simulink model "CE"  (R2021a)
settings: Solver=VariableStepAuto  StartTime=0.0  StopTime=10.0  RelTol=1e-3
(part 1 of 2)
settings Model: Creator=MSI-NB  LastModifiedBy=MSI-NB

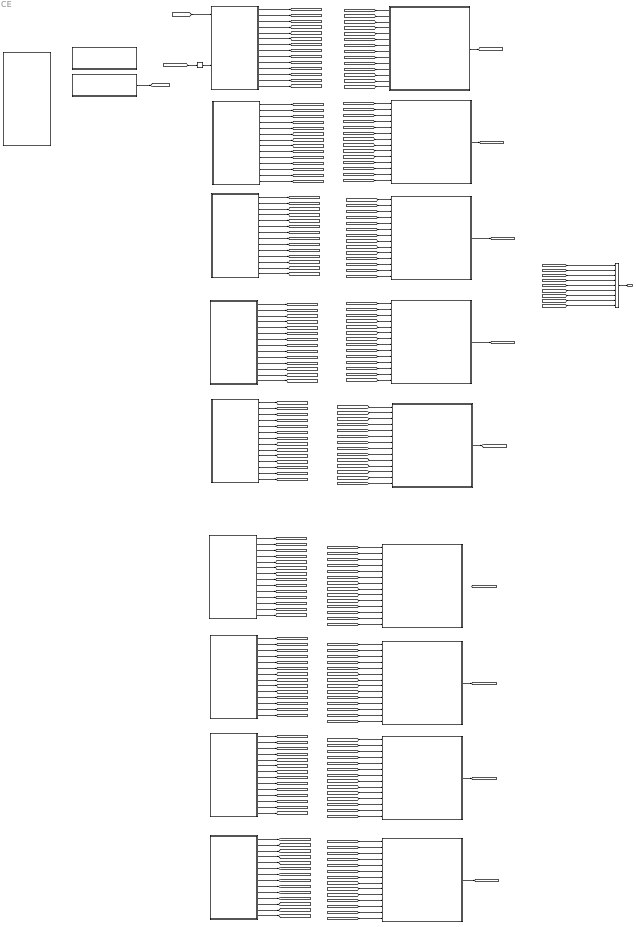
== system CE ==
  Construction : Subsystem
  Construction1 : Subsystem
  ConstructionScenarioCodition : Subsystem
  CruiseOnLane : Subsystem
  CruiseOnLaneScenarioCodition : Subsystem
  Curve : Subsystem
  CurveSenirioConditon : Subsystem
  CutinObjDengerCal : Subsystem
  ILC : Subsystem
  ILCScenarioCodition : Subsystem
  LaneChange : Subsystem
  LaneChangeScenarioCondition : Subsystem
  Memory : Memory
  MergeScenarioCodition : Subsystem
  Min : MinMax  Inputs=9
  Ramp : Subsystem
  RampScenarioCodition : Subsystem
  Split : Subsystem
  SplitScenarioCodition : Subsystem
  TrafficDencity : Subsystem
  Tunnel : Subsystem
  TunnelScenarioCodition : Subsystem
  WrapperCE : Subsystem
  Out1 : Outport
  wires:
  [CruiseOnLaneCE1_2_CE2_Condition] -> CruiseOnLane/1(CruiseOnLaneCE1_2_CE2_Condition)
  [CruiseOnLaneCE1_2_Initial_Condition] -> CruiseOnLane/2(CruiseOnLaneCE1_2_Initial_Condition)
  [CruiseOnLaneCE1_2_CE3_Condition] -> CruiseOnLane/3(CruiseOnLaneCE1_2_CE3_Condition)
  [CruiseOnLaneCE2_2_CE3_Condition] -> CruiseOnLane/4(CruiseOnLaneCE2_2_CE3_Condition)
  [CruiseOnLaneCE2_2_CE1_Condition] -> CruiseOnLane/5(CruiseOnLaneCE2_2_CE1_Condition)
  [CruiseOnLaneCE2_2_Initial_Condition] -> CruiseOnLane/6(CruiseOnLaneCE2_2_Initial_Condition)
  [CruiseOnLaneCE3_2_CE1_Condition] -> CruiseOnLane/7(CruiseOnLaneCE3_2_CE1_Condition)
  [CruiseOnLaneCE3_2_CE2_Condition] -> CruiseOnLane/8(CruiseOnLaneCE3_2_CE2_Condition)
  [CruiseOnLaneCE3_2_Initial_Condition] -> CruiseOnLane/9(CruiseOnLaneCE3_2_Initial_Condition)
  [CruiseOnLaneInitial2CE1_Condition] -> CruiseOnLane/10(CruiseOnLaneInitial2CE1_Condition)
  [CruiseOnLaneInitial2CE2_Condition] -> CruiseOnLane/11(CruiseOnLaneInitial2CE2_Condition)
  [CruiseOnLaneInitial2CE3_Condition] -> CruiseOnLane/12(CruiseOnLaneInitial2CE3_Condition)
  [CruiseOnLaneOFF2ON_Condition] -> CruiseOnLane/13(CruiseOnLaneOFF2ON_Condition)
  [CruiseOnLaneON2OFF_Condition] -> CruiseOnLane/14(CruiseOnLaneON2OFF_Condition)
  [LaneChange_CE1_2_CE2_Condition] -> LaneChange/1(LaneChange_CE1_2_CE2_Condition)
  [LaneChange_CE1_2_Initial_Condition] -> LaneChange/2(LaneChange_CE1_2_Initial_Condition)
  [LaneChange_CE1_2_CE3_Condition] -> LaneChange/3(LaneChange_CE1_2_CE3_Condition)
  [LaneChange_CE2_2_CE3_Condition] -> LaneChange/4(LaneChange_CE2_2_CE3_Condition)
  [LaneChange_CE2_2_CE1_Condition] -> LaneChange/5(LaneChange_CE2_2_CE1_Condition)
  [LaneChange_CE2_2_Initial_Condition] -> LaneChange/6(LaneChange_CE2_2_Initial_Condition)
  [LaneChange_CE3_2_CE1_Condition] -> LaneChange/7(LaneChange_CE3_2_CE1_Condition)
  [LaneChange_CE3_2_CE2_Condition] -> LaneChange/8(LaneChange_CE3_2_CE2_Condition)
  [LaneChange_CE3_2_Initial_Condition] -> LaneChange/9(LaneChange_CE3_2_Initial_Condition)
  [LaneChange_Initial2CE1_Condition] -> LaneChange/10(LaneChange_Initial2CE1_Condition)
  [LaneChange_Initial2CE2_Condition] -> LaneChange/11(LaneChange_Initial2CE2_Condition)
  [LaneChange_Initial2CE3_Condition] -> LaneChange/12(LaneChange_Initial2CE3_Condition)
  [LaneChange_OFF2ON_Condition] -> LaneChange/13(LaneChange_OFF2ON_Condition)
  [LaneChange_ON2OFF_Condition] -> LaneChange/14(LaneChange_ON2OFF_Condition)
  CruiseOnLaneScenarioCodition/1(CruiseOnLaneCE1_2_CE2_Condition) -> [CruiseOnLaneCE1_2_CE2_Condition]  "CruiseOnLaneCE1_2_CE2_Condition"
  CruiseOnLaneScenarioCodition/2(CruiseOnLaneCE1_2_Initial_Condition) -> [CruiseOnLaneCE1_2_Initial_Condition]  "CruiseOnLaneCE1_2_Initial_Condition"
  CruiseOnLaneScenarioCodition/3(CruiseOnLaneCE1_2_CE3_Condition) -> [CruiseOnLaneCE1_2_CE3_Condition]  "CruiseOnLaneCE1_2_CE3_Condition"
  CruiseOnLaneScenarioCodition/4(CruiseOnLaneCE2_2_CE3_Condition) -> [CruiseOnLaneCE2_2_CE3_Condition]  "CruiseOnLaneCE2_2_CE3_Condition"
  CruiseOnLaneScenarioCodition/5(CruiseOnLaneCE2_2_CE1_Condition) -> [CruiseOnLaneCE2_2_CE1_Condition]  "CruiseOnLaneCE2_2_CE1_Condition"
  CruiseOnLaneScenarioCodition/6(CruiseOnLaneCE2_2_Initial_Condition) -> [CruiseOnLaneCE2_2_Initial_Condition]  "CruiseOnLaneCE2_2_Initial_Condition"
  CruiseOnLaneScenarioCodition/7(CruiseOnLaneCE3_2_CE1_Condition) -> [CruiseOnLaneCE3_2_CE1_Condition]  "CruiseOnLaneCE3_2_CE1_Condition"
  CruiseOnLaneScenarioCodition/8(CruiseOnLaneCE3_2_CE2_Condition) -> [CruiseOnLaneCE3_2_CE2_Condition]  "CruiseOnLaneCE3_2_CE2_Condition"
  CruiseOnLaneScenarioCodition/9(CruiseOnLaneCE3_2_Initial_Condition) -> [CruiseOnLaneCE3_2_Initial_Condition]  "CruiseOnLaneCE3_2_Initial_Condition"
  CruiseOnLaneScenarioCodition/10(CruiseOnLaneInitial2CE1_Condition) -> [CruiseOnLaneInitial2CE1_Condition]  "CruiseOnLaneInitial2CE1_Condition"
  CruiseOnLaneScenarioCodition/11(CruiseOnLaneInitial2CE2_Condition) -> [CruiseOnLaneInitial2CE2_Condition]  "CruiseOnLaneInitial2CE2_Condition"
  CruiseOnLaneScenarioCodition/12(CruiseOnLaneInitial2CE3_Condition) -> [CruiseOnLaneInitial2CE3_Condition]  "CruiseOnLaneInitial2CE3_Condition"
  CruiseOnLaneScenarioCodition/13(CruiseOnLaneOFF2ON_Condition) -> [CruiseOnLaneOFF2ON_Condition]  "CruiseOnLaneOFF2ON_Condition"
  CruiseOnLaneScenarioCodition/14(CruiseOnLaneON2OFF_Condition) -> [CruiseOnLaneON2OFF_Condition]  "CruiseOnLaneON2OFF_Condition"
  LaneChangeScenarioCondition/1(LaneChange_CE1_2_CE2_Condition) -> [LaneChange_CE1_2_CE2_Condition]  "LaneChange_CE1_2_CE2_Condition"
  LaneChangeScenarioCondition/2(LaneChange_CE1_2_Initial_Condition) -> [LaneChange_CE1_2_Initial_Condition]  "LaneChange_CE1_2_Initial_Condition"
  LaneChangeScenarioCondition/3(LaneChange_CE1_2_CE3_Condition) -> [LaneChange_CE1_2_CE3_Condition]  "LaneChange_CE1_2_CE3_Condition"
  LaneChangeScenarioCondition/4(LaneChange_CE2_2_CE3_Condition) -> [LaneChange_CE2_2_CE3_Condition]  "LaneChange_CE2_2_CE3_Condition"
  LaneChangeScenarioCondition/5(LaneChange_CE2_2_CE1_Condition) -> [LaneChange_CE2_2_CE1_Condition]  "LaneChange_CE2_2_CE1_Condition"
  LaneChangeScenarioCondition/6(LaneChange_CE2_2_Initial_Condition) -> [LaneChange_CE2_2_Initial_Condition]  "LaneChange_CE2_2_Initial_Condition"
  LaneChangeScenarioCondition/7(LaneChange_CE3_2_CE1_Condition) -> [LaneChange_CE3_2_CE1_Condition]  "LaneChange_CE3_2_CE1_Condition"
  LaneChangeScenarioCondition/8(LaneChange_CE3_2_CE2_Condition) -> [LaneChange_CE3_2_CE2_Condition]  "LaneChange_CE3_2_CE2_Condition"
  LaneChangeScenarioCondition/9(LaneChange_CE3_2_Initial_Condition) -> [LaneChange_CE3_2_Initial_Condition]  "LaneChange_CE3_2_Initial_Condition"
  LaneChangeScenarioCondition/10(LaneChange_Initial2CE1_Condition) -> [LaneChange_Initial2CE1_Condition]  "LaneChange_Initial2CE1_Condition"
  LaneChangeScenarioCondition/11(LaneChange_Initial2CE2_Condition) -> [LaneChange_Initial2CE2_Condition]  "LaneChange_Initial2CE2_Condition"
  LaneChangeScenarioCondition/12(LaneChange_Initial2CE3_Condition) -> [LaneChange_Initial2CE3_Condition]  "LaneChange_Initial2CE3_Condition"
  LaneChangeScenarioCondition/13(LaneChange_OFF2ON_Condition) -> [LaneChange_OFF2ON_Condition]  "LaneChange_OFF2ON_Condition"
  LaneChangeScenarioCondition/14(LaneChange_ON2OFF_Condition) -> [LaneChange_ON2OFF_Condition]  "LaneChange_ON2OFF_Condition"
  Curve/1(CurveConfidenceFlag) -> [CurveConfidenceFlag]  "CurveConfidenceFlag"
  CruiseOnLane/1(CruiseOnLaneConfidenceFlag) -> [CruiseOnLaneConfidenceFlag]
  LaneChange/1(LaneChangeConfidenceFlag) -> [LaneChangeConfidenceFlag]
  Construction/1(ConstructionConfidenceFlag) -> [ConstructionConfidenceFlag]
  ILC/1(ILCConfidenceFlag) -> [ILCConfidenceFlag]
  Ramp/1(RampConfidenceFlag) -> [RampConfidenceFlag]  "RampConfidenceFlag"
  Split/1(SplitConfidenceFlag) -> [SplitConfidenceFlag]
  Tunnel/1(TunnelConfidenceFlag) -> [TunnelConfidenceFlag]
  ConstructionScenarioCodition/1(Construction_CE1_2_CE2_Condition) -> [Construction_CE1_2_CE2_Condition]  "Construction_CE1_2_CE2_Condition"
  ConstructionScenarioCodition/2(Construction_CE1_2_Initial_Condition) -> [Construction_CE1_2_Initial_Condition]  "Construction_CE1_2_Initial_Condition"
  ConstructionScenarioCodition/3(Construction_CE1_2_CE3_Condition) -> [Construction_CE1_2_CE3_Condition]  "Construction_CE1_2_CE3_Condition"
  ConstructionScenarioCodition/4(Construction_CE2_2_CE3_Condition) -> [Construction_CE2_2_CE3_Condition]  "Construction_CE2_2_CE3_Condition"
  ConstructionScenarioCodition/5(Construction_CE2_2_CE1_Condition) -> [Construction_CE2_2_CE1_Condition]  "Construction_CE2_2_CE1_Condition"
  ConstructionScenarioCodition/6(Construction_CE2_2_Initial_Condition) -> [Construction_CE2_2_Initial_Condition]  "Construction_CE2_2_Initial_Condition"
  ConstructionScenarioCodition/7(Construction_CE3_2_CE1_Condition) -> [Construction_CE3_2_CE1_Condition]  "Construction_CE3_2_CE1_Condition"
  ConstructionScenarioCodition/8(Construction_CE3_2_CE2_Condition) -> [Construction_CE3_2_CE2_Condition]  "Construction_CE3_2_CE2_Condition"
  ConstructionScenarioCodition/9(Construction_CE3_2_Initial_Condition) -> [Construction_CE3_2_Initial_Condition]  "Construction_CE3_2_Initial_Condition"
  ConstructionScenarioCodition/10(Construction_Initial2CE1_Condition) -> [Construction_Initial2CE1_Condition]  "Construction_Initial2CE1_Condition"
  ConstructionScenarioCodition/11(Construction_Initial2CE2_Condition) -> [Construction_Initial2CE2_Condition]  "Construction_Initial2CE2_Condition"
  ConstructionScenarioCodition/12(Construction_Initial2CE3_Condition) -> [Construction_Initial2CE3_Condition]  "Construction_Initial2CE3_Condition"
  ConstructionScenarioCodition/13(Construction_OFF2ON_Condition) -> [Construction_OFF2ON_Condition]  "Construction_OFF2ON_Condition"
  ConstructionScenarioCodition/14(Construction_ON2OFF_Condition) -> [Construction_ON2OFF_Condition]  "Construction_ON2OFF_Condition"
  CurveSenirioConditon/1(Curve_CE1_2_CE2_Condition) -> [Curve_CE1_2_CE2_Condition]  "Curve_CE1_2_CE2_Condition"
  CurveSenirioConditon/2(Curve_CE1_2_Initial_Condition) -> [Curve_CE1_2_Initial_Condition]  "Curve_CE1_2_Initial_Condition"
  CurveSenirioConditon/3(Curve_CE1_2_CE3_Condition) -> [Curve_CE1_2_CE3_Condition]  "Curve_CE1_2_CE3_Condition"
  CurveSenirioConditon/4(Curve_CE2_2_CE3_Condition) -> [Curve_CE2_2_CE3_Condition]  "Curve_CE2_2_CE3_Condition"
  CurveSenirioConditon/5(Curve_CE2_2_CE1_Condition) -> [Curve_CE2_2_CE1_Condition]  "Curve_CE2_2_CE1_Condition"
  CurveSenirioConditon/6(Curve_CE2_2_Initial_Condition) -> [Curve_CE2_2_Initial_Condition]  "Curve_CE2_2_Initial_Condition"
  CurveSenirioConditon/7(Curve_CE3_2_CE1_Condition) -> [Curve_CE3_2_CE1_Condition]  "Curve_CE3_2_CE1_Condition"
  CurveSenirioConditon/8(Curve_CE3_2_CE2_Condition) -> [Curve_CE3_2_CE2_Condition]  "Curve_CE3_2_CE2_Condition"
  CurveSenirioConditon/9(Curve_CE3_2_Initial_Condition) -> [Curve_CE3_2_Initial_Condition]  "Curve_CE3_2_Initial_Condition"
  CurveSenirioConditon/10(Curve_Initial2CE1_Condition) -> [Curve_Initial2CE1_Condition]  "Curve_Initial2CE1_Condition"
  CurveSenirioConditon/11(Curve_Initial2CE2_Condition) -> [Curve_Initial2CE2_Condition]  "Curve_Initial2CE2_Condition"
  CurveSenirioConditon/12(Curve_Initial2CE3_Condition) -> [Curve_Initial2CE3_Condition]  "Curve_Initial2CE3_Condition"
  CurveSenirioConditon/13(Curve_OFF2ON_Condition) -> [Curve_OFF2ON_Condition]  "Curve_OFF2ON_Condition"
  CurveSenirioConditon/14(Curve_ON2OFF_Condition) -> [Curve_ON2OFF_Condition]  "Curve_ON2OFF_Condition"
  ILCScenarioCodition/1(ILC_CE1_2_CE2_Condition) -> [ILC_CE1_2_CE2_Condition]  "ILC_CE1_2_CE2_Condition"
  ILCScenarioCodition/2(ILC_CE1_2_Initial_Condition) -> [ILC_CE1_2_Initial_Condition]  "ILC_CE1_2_Initial_Condition"
  ILCScenarioCodition/3(ILC_CE1_2_CE3_Condition) -> [ILC_CE1_2_CE3_Condition]  "ILC_CE1_2_CE3_Condition"
  ILCScenarioCodition/4(ILC_CE2_2_CE3_Condition) -> [ILC_CE2_2_CE3_Condition]  "ILC_CE2_2_CE3_Condition"
  ILCScenarioCodition/5(ILC_CE2_2_CE1_Condition) -> [ILC_CE2_2_CE1_Condition]  "ILC_CE2_2_CE1_Condition"
  ILCScenarioCodition/6(ILC_CE2_2_Initial_Condition) -> [ILC_CE2_2_Initial_Condition]  "ILC_CE2_2_Initial_Condition"
  ILCScenarioCodition/7(ILC_CE3_2_CE1_Condition) -> [ILC_CE3_2_CE1_Condition]  "ILC_CE3_2_CE1_Condition"
  ILCScenarioCodition/8(ILC_CE3_2_CE2_Condition) -> [ILC_CE3_2_CE2_Condition]  "ILC_CE3_2_CE2_Condition"
  ILCScenarioCodition/9(ILC_CE3_2_Initial_Condition) -> [ILC_CE3_2_Initial_Condition]  "ILC_CE3_2_Initial_Condition"
  ILCScenarioCodition/10(ILC_Initial2CE1_Condition) -> [ILC_Initial2CE1_Condition]  "ILC_Initial2CE1_Condition"
  ILCScenarioCodition/11(ILC_Initial2CE2_Condition) -> [ILC_Initial2CE2_Condition]  "ILC_Initial2CE2_Condition"
  ILCScenarioCodition/12(ILC_Initial2CE3_Condition) -> [ILC_Initial2CE3_Condition]  "ILC_Initial2CE3_Condition"
  ILCScenarioCodition/13(ILC_OFF2ON_Condition) -> [ILC_OFF2ON_Condition]  "ILC_OFF2ON_Condition"
  ILCScenarioCodition/14(ILC_ON2OFF_Condition) -> [ILC_ON2OFF_Condition]  "ILC_ON2OFF_Condition"
  MergeScenarioCodition/1(Merge_CE1_2_CE2_Condition) -> [Merge_CE1_2_CE2_Condition]  "Merge_CE1_2_CE2_Condition"
  MergeScenarioCodition/2(Merge_CE1_2_Initial_Condition) -> [Merge_CE1_2_Initial_Condition]  "Merge_CE1_2_Initial_Condition"
  MergeScenarioCodition/3(Merge_CE1_2_CE3_Condition) -> [Merge_CE1_2_CE3_Condition]  "Merge_CE1_2_CE3_Condition"
  MergeScenarioCodition/4(Merge_CE2_2_CE3_Condition) -> [Merge_CE2_2_CE3_Condition]  "Merge_CE2_2_CE3_Condition"
  MergeScenarioCodition/5(Merge_CE2_2_CE1_Condition) -> [Merge_CE2_2_CE1_Condition]  "Merge_CE2_2_CE1_Condition"
  MergeScenarioCodition/6(Merge_CE2_2_Initial_Condition) -> [Merge_CE2_2_Initial_Condition]  "Merge_CE2_2_Initial_Condition"
  MergeScenarioCodition/7(Merge_CE3_2_CE1_Condition) -> [Merge_CE3_2_CE1_Condition]  "Merge_CE3_2_CE1_Condition"
  MergeScenarioCodition/8(Merge_CE3_2_CE2_Condition) -> [Merge_CE3_2_CE2_Condition]  "Merge_CE3_2_CE2_Condition"
  MergeScenarioCodition/9(Merge_CE3_2_Initial_Condition) -> [Merge_CE3_2_Initial_Condition]  "Merge_CE3_2_Initial_Condition"
  MergeScenarioCodition/10(Merge_Initial2CE1_Condition) -> [Merge_Initial2CE1_Condition]  "Merge_Initial2CE1_Condition"
  MergeScenarioCodition/11(Merge_Initial2CE2_Condition) -> [Merge_Initial2CE2_Condition]  "Merge_Initial2CE2_Condition"
  MergeScenarioCodition/12(Merge_Initial2CE3_Condition) -> [Merge_Initial2CE3_Condition]  "Merge_Initial2CE3_Condition"
  MergeScenarioCodition/13(Merge_OFF2ON_Condition) -> [Merge_OFF2ON_Condition]  "Merge_OFF2ON_Condition"
  MergeScenarioCodition/14(Merge_ON2OFF_Condition) -> [Merge_ON2OFF_Condition]  "Merge_ON2OFF_Condition"
  RampScenarioCodition/1(Ramp_CE1_2_CE2_Condition) -> [Ramp_CE1_2_CE2_Condition]  "Ramp_CE1_2_CE2_Condition"
  RampScenarioCodition/2(Ramp_CE1_2_Initial_Condition) -> [Ramp_CE1_2_Initial_Condition]  "Ramp_CE1_2_Initial_Condition"
  RampScenarioCodition/3(Ramp_CE1_2_CE3_Condition) -> [Ramp_CE1_2_CE3_Condition]  "Ramp_CE1_2_CE3_Condition"
  RampScenarioCodition/4(Ramp_CE2_2_CE3_Condition) -> [Ramp_CE2_2_CE3_Condition]  "Ramp_CE2_2_CE3_Condition"
  RampScenarioCodition/5(Ramp_CE2_2_CE1_Condition) -> [Ramp_CE2_2_CE1_Condition]  "Ramp_CE2_2_CE1_Condition"
  RampScenarioCodition/6(Ramp_CE2_2_Initial_Condition) -> [Ramp_CE2_2_Initial_Condition]  "Ramp_CE2_2_Initial_Condition"
  RampScenarioCodition/7(Ramp_CE3_2_CE1_Condition) -> [Ramp_CE3_2_CE1_Condition]  "Ramp_CE3_2_CE1_Condition"
  RampScenarioCodition/8(Ramp_CE3_2_CE2_Condition) -> [Ramp_CE3_2_CE2_Condition]  "Ramp_CE3_2_CE2_Condition"
  RampScenarioCodition/9(Ramp_CE3_2_Initial_Condition) -> [Ramp_CE3_2_Initial_Condition]  "Ramp_CE3_2_Initial_Condition"
  RampScenarioCodition/10(Ramp_Initial2CE1_Condition) -> [Ramp_Initial2CE1_Condition]  "Ramp_Initial2CE1_Condition"
  RampScenarioCodition/11(Ramp_Initial2CE2_Condition) -> [Ramp_Initial2CE2_Condition]  "Ramp_Initial2CE2_Condition"
  RampScenarioCodition/12(Ramp_Initial2CE3_Condition) -> [Ramp_Initial2CE3_Condition]  "Ramp_Initial2CE3_Condition"
  RampScenarioCodition/13(Ramp_OFF2ON_Condition) -> [Ramp_OFF2ON_Condition]  "Ramp_OFF2ON_Condition"
  RampScenarioCodition/14(Ramp_ON2OFF_Condition) -> [Ramp_ON2OFF_Condition]  "Ramp_ON2OFF_Condition"
  SplitScenarioCodition/1(Split_CE1_2_CE2_Condition) -> [Split_CE1_2_CE2_Condition]  "Split_CE1_2_CE2_Condition"
  SplitScenarioCodition/2(Split_CE1_2_Initial_Condition) -> [Split_CE1_2_Initial_Condition]  "Split_CE1_2_Initial_Condition"
  SplitScenarioCodition/3(Split_CE1_2_CE3_Condition) -> [Split_CE1_2_CE3_Condition]  "Split_CE1_2_CE3_Condition"
  SplitScenarioCodition/4(Split_CE2_2_CE3_Condition) -> [Split_CE2_2_CE3_Condition]  "Split_CE2_2_CE3_Condition"
  SplitScenarioCodition/5(Split_CE2_2_CE1_Condition) -> [Split_CE2_2_CE1_Condition]  "Split_CE2_2_CE1_Condition"
  SplitScenarioCodition/6(Split_CE2_2_Initial_Condition) -> [Split_CE2_2_Initial_Condition]  "Split_CE2_2_Initial_Condition"
  SplitScenarioCodition/7(Split_CE3_2_CE1_Condition) -> [Split_CE3_2_CE1_Condition]  "Split_CE3_2_CE1_Condition"
  SplitScenarioCodition/8(Split_CE3_2_CE2_Condition) -> [Split_CE3_2_CE2_Condition]  "Split_CE3_2_CE2_Condition"
  SplitScenarioCodition/9(Split_CE3_2_Initial_Condition) -> [Split_CE3_2_Initial_Condition]  "Split_CE3_2_Initial_Condition"
  SplitScenarioCodition/10(Split_Initial2CE1_Condition) -> [Split_Initial2CE1_Condition]  "Split_Initial2CE1_Condition"
  SplitScenarioCodition/11(Split_Initial2CE2_Condition) -> [Split_Initial2CE2_Condition]  "Split_Initial2CE2_Condition"
  SplitScenarioCodition/12(Split_Initial2CE3_Condition) -> [Split_Initial2CE3_Condition]  "Split_Initial2CE3_Condition"
  SplitScenarioCodition/13(Split_OFF2ON_Condition) -> [Split_OFF2ON_Condition]  "Split_OFF2ON_Condition"
  SplitScenarioCodition/14(Split_ON2OFF_Condition) -> [Split_ON2OFF_Condition]  "Split_ON2OFF_Condition"
  TunnelScenarioCodition/1(Tunnel_CE1_2_CE2_Condition) -> [Tunnel_CE1_2_CE2_Condition]  "Tunnel_CE1_2_CE2_Condition"
  TunnelScenarioCodition/2(Tunnel_CE1_2_Initial_Condition) -> [Tunnel_CE1_2_Initial_Condition]  "Tunnel_CE1_2_Initial_Condition"
  TunnelScenarioCodition/3(Tunnel_CE1_2_CE3_Condition) -> [Tunnel_CE1_2_CE3_Condition]  "Tunnel_CE1_2_CE3_Condition"
  TunnelScenarioCodition/4(Tunnel_CE2_2_CE3_Condition) -> [Tunnel_CE2_2_CE3_Condition]  "Tunnel_CE2_2_CE3_Condition"
  TunnelScenarioCodition/5(Tunnel_CE2_2_CE1_Condition) -> [Tunnel_CE2_2_CE1_Condition]  "Tunnel_CE2_2_CE1_Condition"
  TunnelScenarioCodition/6(Tunnel_CE2_2_Initial_Condition) -> [Tunnel_CE2_2_Initial_Condition]  "Tunnel_CE2_2_Initial_Condition"
  TunnelScenarioCodition/7(Tunnel_CE3_2_CE1_Condition) -> [Tunnel_CE3_2_CE1_Condition]  "Tunnel_CE3_2_CE1_Condition"
  TunnelScenarioCodition/8(Tunnel_CE3_2_CE2_Condition) -> [Tunnel_CE3_2_CE2_Condition]  "Tunnel_CE3_2_CE2_Condition"
  TunnelScenarioCodition/9(Tunnel_CE3_2_Initial_Condition) -> [Tunnel_CE3_2_Initial_Condition]  "Tunnel_CE3_2_Initial_Condition"
  TunnelScenarioCodition/10(Tunnel_Initial2CE1_Condition) -> [Tunnel_Initial2CE1_Condition]  "Tunnel_Initial2CE1_Condition"
  TunnelScenarioCodition/11(Tunnel_Initial2CE2_Condition) -> [Tunnel_Initial2CE2_Condition]  "Tunnel_Initial2CE2_Condition"
  TunnelScenarioCodition/12(Tunnel_Initial2CE3_Condition) -> [Tunnel_Initial2CE3_Condition]  "Tunnel_Initial2CE3_Condition"
  TunnelScenarioCodition/13(Tunnel_OFF2ON_Condition) -> [Tunnel_OFF2ON_Condition]  "Tunnel_OFF2ON_Condition"
  TunnelScenarioCodition/14(LaneChange_ON2OFF_Condition) -> [Tunnel_ON2OFF_Condition]  "LaneChange_ON2OFF_Condition"
  [Curve_CE2_2_Initial_Condition] -> Curve/6(CE2_2_Initial_Condition)
  [Curve_CE3_2_Initial_Condition] -> Curve/9(CE3_2_Initial_Condition)
  [Curve_CE1_2_Initial_Condition] -> Curve/2(CE1_2_Initial_Condition)
  [Curve_Initial2CE2_Condition] -> Curve/11(Initial2CE2_Condition)
  [Curve_Initial2CE1_Condition] -> Curve/10(Initial2CE1_Condition)
  [Curve_CE2_2_CE3_Condition] -> Curve/4(CE2_2_CE3_Condition)
  [Curve_CE2_2_CE1_Condition] -> Curve/5(CE2_2_CE1_Condition)
  [Curve_CE3_2_CE1_Condition] -> Curve/7(CE3_2_CE1_Condition)
  [Curve_CE3_2_CE2_Condition] -> Curve/8(CE3_2_CE2_Condition)
  [Curve_CE1_2_CE2_Condition] -> Curve/1(CE1_2_CE2_Condition)
  [Curve_CE1_2_CE3_Condition] -> Curve/3(CE1_2_CE3_Condition)
  [Curve_Initial2CE3_Condition] -> Curve/12(Initial2CE3_Condition)
  [Curve_OFF2ON_Condition] -> Curve/13(OFF2ON_Condition)
  [Curve_ON2OFF_Condition] -> Curve/14(ON2OFF_Condition)
  [Ramp_CE1_2_Initial_Condition] -> Ramp/2(CE1_2_Initial_Condition)
  [Ramp_CE2_2_Initial_Condition] -> Ramp/6(CE2_2_Initial_Condition)
  [Ramp_CE3_2_Initial_Condition] -> Ramp/9(CE3_2_Initial_Condition)
  [Ramp_Initial2CE1_Condition] -> Ramp/10(Initial2CE1_Condition)
  [Ramp_Initial2CE2_Condition] -> Ramp/11(Initial2CE2_Condition)
  [Ramp_Initial2CE3_Condition] -> Ramp/12(Initial2CE3_Condition)
  [Ramp_CE1_2_CE2_Condition] -> Ramp/1(CE1_2_CE2_Condition)
  [Ramp_CE1_2_CE3_Condition] -> Ramp/3(CE1_2_CE3_Condition)
  [Ramp_CE2_2_CE3_Condition] -> Ramp/4(CE2_2_CE3_Condition)
  [Ramp_CE2_2_CE1_Condition] -> Ramp/5(CE2_2_CE1_Condition)
  [Ramp_CE3_2_CE1_Condition] -> Ramp/7(CE3_2_CE1_Condition)
  [Ramp_CE3_2_CE2_Condition] -> Ramp/8(CE3_2_CE2_Condition)
  [Ramp_OFF2ON_Condition] -> Ramp/13(OFF2ON_Condition)
  [Ramp_ON2OFF_Condition] -> Ramp/14(ON2OFF_Condition)
  [Split_CE1_2_Initial_Condition] -> Split/2(CE1_2_Initial_Condition)
  [Split_CE2_2_Initial_Condition] -> Split/6(CE2_2_Initial_Condition)
  [Split_CE3_2_Initial_Condition] -> Split/9(CE3_2_Initial_Condition)
  [Split_Initial2CE1_Condition] -> Split/10(Initial2CE1_Condition)
  [Split_Initial2CE2_Condition] -> Split/11(Initial2CE2_Condition)
  [Split_Initial2CE3_Condition] -> Split/12(Initial2CE3_Condition)
  [Split_CE1_2_CE2_Condition] -> Split/1(CE1_2_CE2_Condition)
  [Split_CE1_2_CE3_Condition] -> Split/3(CE1_2_CE3_Condition)
  [Split_CE2_2_CE3_Condition] -> Split/4(CE2_2_CE3_Condition)
  [Split_CE2_2_CE1_Condition] -> Split/5(CE2_2_CE1_Condition)
  [Split_CE3_2_CE1_Condition] -> Split/7(CE3_2_CE1_Condition)
  [Split_CE3_2_CE2_Condition] -> Split/8(CE3_2_CE2_Condition)
  [Split_OFF2ON_Condition] -> Split/13(OFF2ON_Condition)
  [Split_ON2OFF_Condition] -> Split/14(ON2OFF_Condition)
  [Construction_CE1_2_Initial_Condition] -> Construction1/2(CE1_2_Initial_Condition)
  [Construction_CE2_2_Initial_Condition] -> Construction1/6(CE2_2_Initial_Condition)
  [Construction_CE3_2_Initial_Condition] -> Construction1/9(CE3_2_Initial_Condition)
  [Construction_Initial2CE1_Condition] -> Construction1/10(Initial2CE1_Condition)
  [Construction_Initial2CE2_Condition] -> Construction1/11(Initial2CE2_Condition)
  [Construction_Initial2CE3_Condition] -> Construction1/12(Initial2CE3_Condition)
  [Construction_ON2OFF_Condition] -> Construction1/14(ON2OFF_Condition)
  [Construction_CE1_2_CE2_Condition] -> Construction1/1(CE1_2_CE2_Condition)
  [Construction_CE1_2_CE3_Condition] -> Construction1/3(CE1_2_CE3_Condition)
  [Construction_CE2_2_CE3_Condition] -> Construction1/4(CE2_2_CE3_Condition)
  [Construction_CE2_2_CE1_Condition] -> Construction1/5(CE2_2_CE1_Condition)
  [Construction_CE3_2_CE1_Condition] -> Construction1/7(CE3_2_CE1_Condition)
  [Construction_CE3_2_CE2_Condition] -> Construction1/8(CE3_2_CE2_Condition)
  [Construction_OFF2ON_Condition] -> Construction1/13(OFF2ON_Condition)
  [Tunnel_CE3_2_Initial_Condition] -> ILC/9(CE3_2_Initial_Condition)
  [Tunnel_Initial2CE1_Condition] -> ILC/10(Initial2CE1_Condition)
  [Tunnel_Initial2CE2_Condition] -> ILC/11(Initial2CE2_Condition)
  [Tunnel_Initial2CE3_Condition] -> ILC/12(Initial2CE3_Condition)
  [Tunnel_CE1_2_Initial_Condition] -> ILC/2(CE1_2_Initial_Condition)
  [Tunnel_CE2_2_Initial_Condition] -> ILC/6(CE2_2_Initial_Condition)
  [Tunnel_ON2OFF_Condition] -> ILC/14(ON2OFF_Condition)
  [Tunnel_CE1_2_CE2_Condition] -> ILC/1(CE1_2_CE2_Condition)
  [Tunnel_CE1_2_CE3_Condition] -> ILC/3(CE1_2_CE3_Condition)
  [Tunnel_CE2_2_CE3_Condition] -> ILC/4(CE2_2_CE3_Condition)
  [Tunnel_CE2_2_CE1_Condition] -> ILC/5(CE2_2_CE1_Condition)
  [Tunnel_CE3_2_CE1_Condition] -> ILC/7(CE3_2_CE1_Condition)
  [Tunnel_CE3_2_CE2_Condition] -> ILC/8(CE3_2_CE2_Condition)
  [Tunnel_OFF2ON_Condition] -> ILC/13(OFF2ON_Condition)
  [Merge_CE1_2_Initial_Condition] -> Tunnel/2(CE1_2_Initial_Condition)
  [Merge_CE2_2_Initial_Condition] -> Tunnel/6(CE2_2_Initial_Condition)
  [Merge_CE3_2_Initial_Condition] -> Tunnel/9(CE3_2_Initial_Condition)
  [Merge_Initial2CE1_Condition] -> Tunnel/10(Initial2CE1_Condition)
  [Merge_Initial2CE2_Condition] -> Tunnel/11(Initial2CE2_Condition)
  [Merge_Initial2CE3_Condition] -> Tunnel/12(Initial2CE3_Condition)
  [Merge_CE1_2_CE2_Condition] -> Tunnel/1(CE1_2_CE2_Condition)
  [Merge_CE1_2_CE3_Condition] -> Tunnel/3(CE1_2_CE3_Condition)
  [Merge_CE2_2_CE3_Condition] -> Tunnel/4(CE2_2_CE3_Condition)
  [Merge_CE2_2_CE1_Condition] -> Tunnel/5(CE2_2_CE1_Condition)
  [Merge_CE3_2_CE1_Condition] -> Tunnel/7(CE3_2_CE1_Condition)
  [Merge_CE3_2_CE2_Condition] -> Tunnel/8(CE3_2_CE2_Condition)
  [Merge_OFF2ON_Condition] -> Tunnel/13(OFF2ON_Condition)
  [Merge_ON2OFF_Condition] -> Tunnel/14(ON2OFF_Condition)
  [ILC_CE1_2_Initial_Condition] -> Construction/2(CE1_2_Initial_Condition)
  [ILC_CE2_2_Initial_Condition] -> Construction/6(CE2_2_Initial_Condition)
  [ILC_CE3_2_Initial_Condition] -> Construction/9(CE3_2_Initial_Condition)
  [ILC_Initial2CE1_Condition] -> Construction/10(Initial2CE1_Condition)
  [ILC_Initial2CE2_Condition] -> Construction/11(Initial2CE2_Condition)
  [ILC_Initial2CE3_Condition] -> Construction/12(Initial2CE3_Condition)
  [ILC_CE1_2_CE2_Condition] -> Construction/1(CE1_2_CE2_Condition)
  [ILC_CE1_2_CE3_Condition] -> Construction/3(CE1_2_CE3_Condition)
  [ILC_CE2_2_CE3_Condition] -> Construction/4(CE2_2_CE3_Condition)
  [ILC_CE2_2_CE1_Condition] -> Construction/5(CE2_2_CE1_Condition)
  [ILC_CE3_2_CE1_Condition] -> Construction/7(CE3_2_CE1_Condition)
  [ILC_CE3_2_CE2_Condition] -> Construction/8(CE3_2_CE2_Condition)
  [ILC_OFF2ON_Condition] -> Construction/13(OFF2ON_Condition)
  [ILC_ON2OFF_Condition] -> Construction/14(ON2OFF_Condition)
  [ConstructionConfidenceFlag] -> Min/9
  [TunnelConfidenceFlag] -> Min/8
  [ILCConfidenceFlag] -> Min/7
  [MergeConfidenceFlag] -> Min/6
  [SplitConfidenceFlag] -> Min/5
  [RampConfidenceFlag] -> Min/4
  [CurveConfidenceFlag] -> Min/3
  [LaneChangeConfidenceFlag] -> Min/2
  [CruiseOnLaneConfidenceFlag] -> Min/1
  Min/1 -> Out1/1
  CutinObjDengerCal/1(CutinDengerTarget) -> [CutinTarget]
  [CutinTarget] -> CruiseOnLaneScenarioCodition/1(CutinTarget)  "CutinTarget"
  [CruiseOnLaneConfidenceFlag] -> Memory/1  "CruiseOnLaneConfidenceFlag"
  Memory/1 -> CruiseOnLaneScenarioCodition/4(CruiseOnLaneConfidenceFlagPrev)

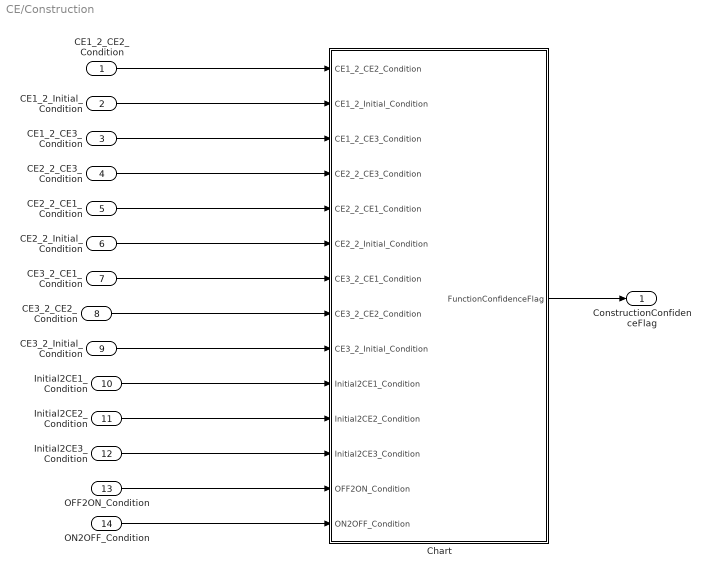
== system CE/Construction ==
  CE1_2_CE2_Condition : Inport
  CE1_2_Initial_Condition : Inport  Port=2
  CE1_2_CE3_Condition : Inport  Port=3
  CE2_2_CE3_Condition : Inport  Port=4
  CE2_2_CE1_Condition : Inport  Port=5
  CE2_2_Initial_Condition : Inport  Port=6
  CE3_2_CE1_Condition : Inport  Port=7
  CE3_2_CE2_Condition : Inport  Port=8
  CE3_2_Initial_Condition : Inport  Port=9
  Initial2CE1_Condition : Inport  Port=10
  Initial2CE2_Condition : Inport  Port=11
  Initial2CE3_Condition : Inport  Port=12
  OFF2ON_Condition : Inport  Port=13
  ON2OFF_Condition : Inport  Port=14
  Chart : Stateflow chart  TreatAsAtomicUnit=on
  ConstructionConfidenceFlag : Outport
  wires:
  Chart/1(FunctionConfidenceFlag) -> ConstructionConfidenceFlag/1
  CE1_2_CE2_Condition/1 -> Chart/1(CE1_2_CE2_Condition)
  CE1_2_Initial_Condition/1 -> Chart/2(CE1_2_Initial_Condition)
  CE1_2_CE3_Condition/1 -> Chart/3(CE1_2_CE3_Condition)
  CE2_2_CE3_Condition/1 -> Chart/4(CE2_2_CE3_Condition)
  CE2_2_CE1_Condition/1 -> Chart/5(CE2_2_CE1_Condition)
  CE2_2_Initial_Condition/1 -> Chart/6(CE2_2_Initial_Condition)
  CE3_2_CE1_Condition/1 -> Chart/7(CE3_2_CE1_Condition)
  CE3_2_CE2_Condition/1 -> Chart/8(CE3_2_CE2_Condition)
  CE3_2_Initial_Condition/1 -> Chart/9(CE3_2_Initial_Condition)
  Initial2CE1_Condition/1 -> Chart/10(Initial2CE1_Condition)
  Initial2CE2_Condition/1 -> Chart/11(Initial2CE2_Condition)
  Initial2CE3_Condition/1 -> Chart/12(Initial2CE3_Condition)
  OFF2ON_Condition/1 -> Chart/13(OFF2ON_Condition)
  ON2OFF_Condition/1 -> Chart/14(ON2OFF_Condition)

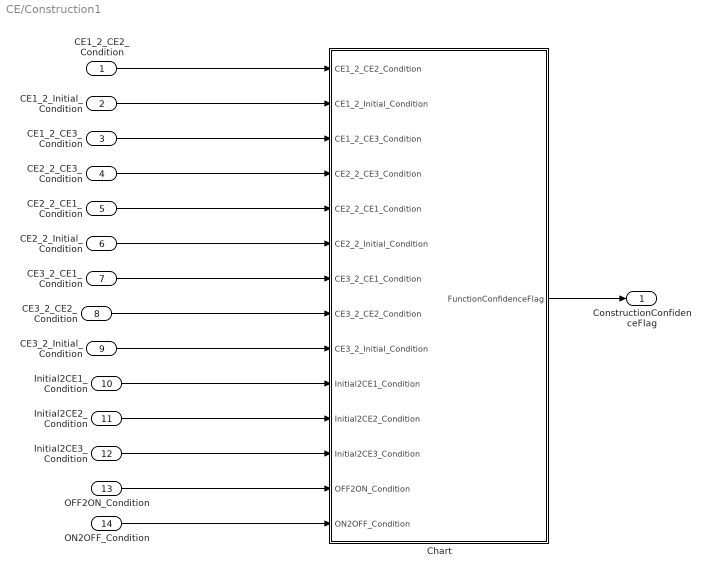
== system CE/Construction1 ==
  CE1_2_CE2_Condition : Inport
  CE1_2_Initial_Condition : Inport  Port=2
  CE1_2_CE3_Condition : Inport  Port=3
  CE2_2_CE3_Condition : Inport  Port=4
  CE2_2_CE1_Condition : Inport  Port=5
  CE2_2_Initial_Condition : Inport  Port=6
  CE3_2_CE1_Condition : Inport  Port=7
  CE3_2_CE2_Condition : Inport  Port=8
  CE3_2_Initial_Condition : Inport  Port=9
  Initial2CE1_Condition : Inport  Port=10
  Initial2CE2_Condition : Inport  Port=11
  Initial2CE3_Condition : Inport  Port=12
  OFF2ON_Condition : Inport  Port=13
  ON2OFF_Condition : Inport  Port=14
  Chart : Stateflow chart  TreatAsAtomicUnit=on
  ConstructionConfidenceFlag : Outport
  wires:
  ON2OFF_Condition/1 -> Chart/14(ON2OFF_Condition)
  OFF2ON_Condition/1 -> Chart/13(OFF2ON_Condition)
  Initial2CE3_Condition/1 -> Chart/12(Initial2CE3_Condition)
  Initial2CE2_Condition/1 -> Chart/11(Initial2CE2_Condition)
  Initial2CE1_Condition/1 -> Chart/10(Initial2CE1_Condition)
  CE3_2_Initial_Condition/1 -> Chart/9(CE3_2_Initial_Condition)
  CE3_2_CE2_Condition/1 -> Chart/8(CE3_2_CE2_Condition)
  CE3_2_CE1_Condition/1 -> Chart/7(CE3_2_CE1_Condition)
  CE2_2_Initial_Condition/1 -> Chart/6(CE2_2_Initial_Condition)
  CE2_2_CE1_Condition/1 -> Chart/5(CE2_2_CE1_Condition)
  CE2_2_CE3_Condition/1 -> Chart/4(CE2_2_CE3_Condition)
  CE1_2_CE3_Condition/1 -> Chart/3(CE1_2_CE3_Condition)
  CE1_2_Initial_Condition/1 -> Chart/2(CE1_2_Initial_Condition)
  CE1_2_CE2_Condition/1 -> Chart/1(CE1_2_CE2_Condition)
  Chart/1(FunctionConfidenceFlag) -> ConstructionConfidenceFlag/1

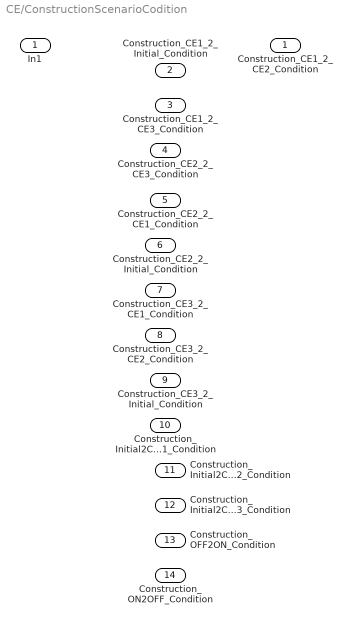
== system CE/ConstructionScenarioCodition ==
  In1 : Inport
  Construction_CE1_2_CE2_Condition : Outport
  Construction_CE1_2_Initial_Condition : Outport  Port=2
  Construction_CE1_2_CE3_Condition : Outport  Port=3
  Construction_CE2_2_CE3_Condition : Outport  Port=4
  Construction_CE2_2_CE1_Condition : Outport  Port=5
  Construction_CE2_2_Initial_Condition : Outport  Port=6
  Construction_CE3_2_CE1_Condition : Outport  Port=7
  Construction_CE3_2_CE2_Condition : Outport  Port=8
  Construction_CE3_2_Initial_Condition : Outport  Port=9
  Construction_Initial2CE1_Condition : Outport  Port=10
  Construction_Initial2CE2_Condition : Outport  Port=11
  Construction_Initial2CE3_Condition : Outport  Port=12
  Construction_OFF2ON_Condition : Outport  Port=13
  Construction_ON2OFF_Condition : Outport  Port=14

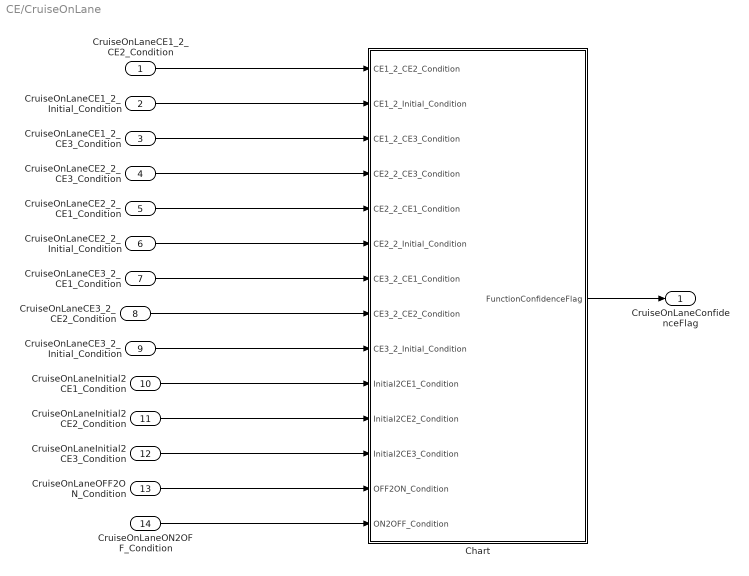
== system CE/CruiseOnLane ==
  CruiseOnLaneCE1_2_CE2_Condition : Inport
  CruiseOnLaneCE1_2_Initial_Condition : Inport  Port=2
  CruiseOnLaneCE1_2_CE3_Condition : Inport  Port=3
  CruiseOnLaneCE2_2_CE3_Condition : Inport  Port=4
  CruiseOnLaneCE2_2_CE1_Condition : Inport  Port=5
  CruiseOnLaneCE2_2_Initial_Condition : Inport  Port=6
  CruiseOnLaneCE3_2_CE1_Condition : Inport  Port=7
  CruiseOnLaneCE3_2_CE2_Condition : Inport  Port=8
  CruiseOnLaneCE3_2_Initial_Condition : Inport  Port=9
  CruiseOnLaneInitial2CE1_Condition : Inport  Port=10
  CruiseOnLaneInitial2CE2_Condition : Inport  Port=11
  CruiseOnLaneInitial2CE3_Condition : Inport  Port=12
  CruiseOnLaneOFF2ON_Condition : Inport  Port=13
  CruiseOnLaneON2OFF_Condition : Inport  Port=14
  Chart : Stateflow chart  TreatAsAtomicUnit=on
  CruiseOnLaneConfidenceFlag : Outport
  wires:
  Chart/1(FunctionConfidenceFlag) -> CruiseOnLaneConfidenceFlag/1
  CruiseOnLaneCE1_2_CE2_Condition/1 -> Chart/1(CE1_2_CE2_Condition)
  CruiseOnLaneCE1_2_Initial_Condition/1 -> Chart/2(CE1_2_Initial_Condition)
  CruiseOnLaneCE1_2_CE3_Condition/1 -> Chart/3(CE1_2_CE3_Condition)
  CruiseOnLaneCE2_2_CE3_Condition/1 -> Chart/4(CE2_2_CE3_Condition)
  CruiseOnLaneCE2_2_CE1_Condition/1 -> Chart/5(CE2_2_CE1_Condition)
  CruiseOnLaneCE2_2_Initial_Condition/1 -> Chart/6(CE2_2_Initial_Condition)
  CruiseOnLaneCE3_2_CE1_Condition/1 -> Chart/7(CE3_2_CE1_Condition)
  CruiseOnLaneCE3_2_CE2_Condition/1 -> Chart/8(CE3_2_CE2_Condition)
  CruiseOnLaneCE3_2_Initial_Condition/1 -> Chart/9(CE3_2_Initial_Condition)
  CruiseOnLaneInitial2CE1_Condition/1 -> Chart/10(Initial2CE1_Condition)
  CruiseOnLaneInitial2CE2_Condition/1 -> Chart/11(Initial2CE2_Condition)
  CruiseOnLaneInitial2CE3_Condition/1 -> Chart/12(Initial2CE3_Condition)
  CruiseOnLaneOFF2ON_Condition/1 -> Chart/13(OFF2ON_Condition)
  CruiseOnLaneON2OFF_Condition/1 -> Chart/14(ON2OFF_Condition)

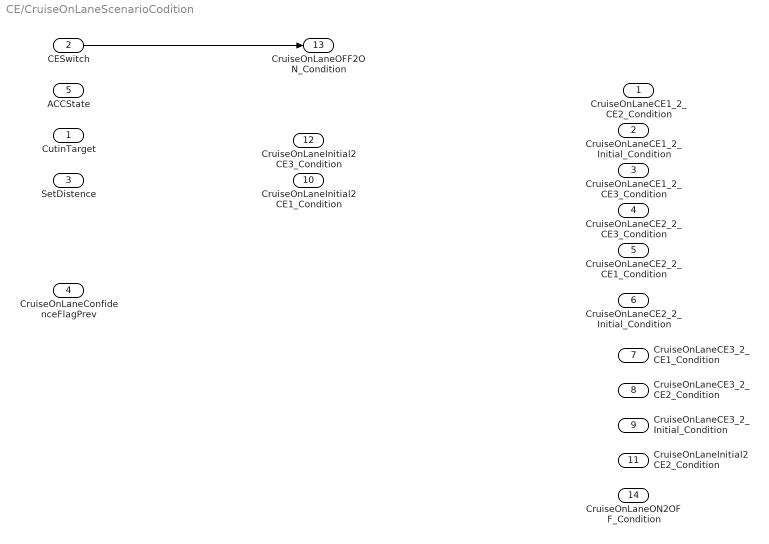
== system CE/CruiseOnLaneScenarioCodition ==
  CutinTarget : Inport
  CESwitch : Inport  Port=2
  SetDistence : Inport  Port=3
  CruiseOnLaneConfidenceFlagPrev : Inport  Port=4
  ACCState : Inport  Port=5
  CruiseOnLaneCE1_2_CE2_Condition : Outport
  CruiseOnLaneCE1_2_Initial_Condition : Outport  Port=2
  CruiseOnLaneCE1_2_CE3_Condition : Outport  Port=3
  CruiseOnLaneCE2_2_CE3_Condition : Outport  Port=4
  CruiseOnLaneCE2_2_CE1_Condition : Outport  Port=5
  CruiseOnLaneCE2_2_Initial_Condition : Outport  Port=6
  CruiseOnLaneCE3_2_CE1_Condition : Outport  Port=7
  CruiseOnLaneCE3_2_CE2_Condition : Outport  Port=8
  CruiseOnLaneCE3_2_Initial_Condition : Outport  Port=9
  CruiseOnLaneInitial2CE1_Condition : Outport  Port=10
  CruiseOnLaneInitial2CE2_Condition : Outport  Port=11
  CruiseOnLaneInitial2CE3_Condition : Outport  Port=12
  CruiseOnLaneOFF2ON_Condition : Outport  Port=13
  CruiseOnLaneON2OFF_Condition : Outport  Port=14
  wires:
  CESwitch/1 -> CruiseOnLaneOFF2ON_Condition/1

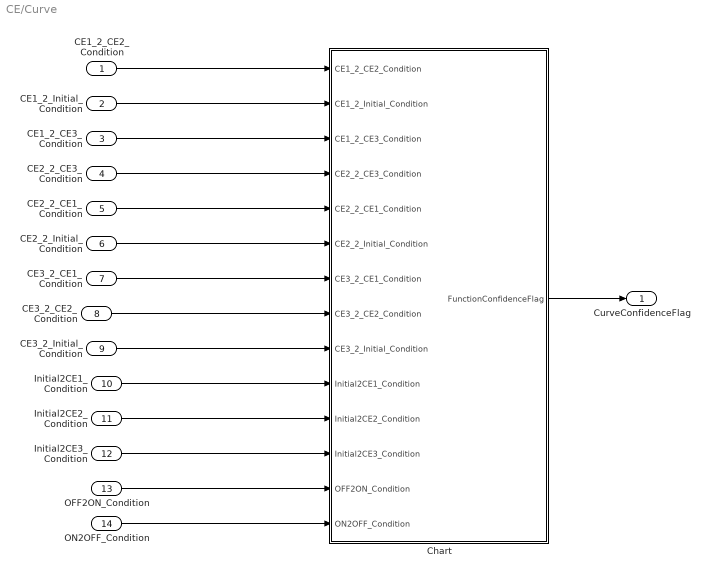
== system CE/Curve ==
  CE1_2_CE2_Condition : Inport
  CE1_2_Initial_Condition : Inport  Port=2
  CE1_2_CE3_Condition : Inport  Port=3
  CE2_2_CE3_Condition : Inport  Port=4
  CE2_2_CE1_Condition : Inport  Port=5
  CE2_2_Initial_Condition : Inport  Port=6
  CE3_2_CE1_Condition : Inport  Port=7
  CE3_2_CE2_Condition : Inport  Port=8
  CE3_2_Initial_Condition : Inport  Port=9
  Initial2CE1_Condition : Inport  Port=10
  Initial2CE2_Condition : Inport  Port=11
  Initial2CE3_Condition : Inport  Port=12
  OFF2ON_Condition : Inport  Port=13
  ON2OFF_Condition : Inport  Port=14
  Chart : Stateflow chart  TreatAsAtomicUnit=on
  CurveConfidenceFlag : Outport
  wires:
  Chart/1(FunctionConfidenceFlag) -> CurveConfidenceFlag/1
  CE1_2_CE2_Condition/1 -> Chart/1(CE1_2_CE2_Condition)
  CE1_2_Initial_Condition/1 -> Chart/2(CE1_2_Initial_Condition)
  CE1_2_CE3_Condition/1 -> Chart/3(CE1_2_CE3_Condition)
  CE2_2_CE3_Condition/1 -> Chart/4(CE2_2_CE3_Condition)
  CE2_2_CE1_Condition/1 -> Chart/5(CE2_2_CE1_Condition)
  CE2_2_Initial_Condition/1 -> Chart/6(CE2_2_Initial_Condition)
  CE3_2_CE1_Condition/1 -> Chart/7(CE3_2_CE1_Condition)
  CE3_2_CE2_Condition/1 -> Chart/8(CE3_2_CE2_Condition)
  CE3_2_Initial_Condition/1 -> Chart/9(CE3_2_Initial_Condition)
  Initial2CE1_Condition/1 -> Chart/10(Initial2CE1_Condition)
  Initial2CE2_Condition/1 -> Chart/11(Initial2CE2_Condition)
  Initial2CE3_Condition/1 -> Chart/12(Initial2CE3_Condition)
  OFF2ON_Condition/1 -> Chart/13(OFF2ON_Condition)
  ON2OFF_Condition/1 -> Chart/14(ON2OFF_Condition)

== system CE/CurveSenirioConditon ==
  In1 : Inport
  Curve_CE1_2_CE2_Condition : Outport
  Curve_CE1_2_Initial_Condition : Outport  Port=2
  Curve_CE1_2_CE3_Condition : Outport  Port=3
  Curve_CE2_2_CE3_Condition : Outport  Port=4
  Curve_CE2_2_CE1_Condition : Outport  Port=5
  Curve_CE2_2_Initial_Condition : Outport  Port=6
  Curve_CE3_2_CE1_Condition : Outport  Port=7
  Curve_CE3_2_CE2_Condition : Outport  Port=8
  Curve_CE3_2_Initial_Condition : Outport  Port=9
  Curve_Initial2CE1_Condition : Outport  Port=10
  Curve_Initial2CE2_Condition : Outport  Port=11
  Curve_Initial2CE3_Condition : Outport  Port=12
  Curve_OFF2ON_Condition : Outport  Port=13
  Curve_ON2OFF_Condition : Outport  Port=14

== system CE/CutinObjDengerCal ==
  CutinTarget_ID : Inport
  SDF_Object : Inport  Port=2
  Constant : Constant
  CutinTargetSearch : Stateflow chart  TreatAsAtomicUnit=on
  CutinDengerTarget : Outport
  wires:
  CutinTarget_ID/1 -> CutinTargetSearch/2(CutinTarget_ID)  "CutinTarget_ID"
  SDF_Object/1 -> CutinTargetSearch/3(SDF_Object)  "SDF_Object"
  Constant/1 -> CutinTargetSearch/1(OBJ_VD_ZERO)
  CutinTargetSearch/1(CutinTarget) -> CutinDengerTarget/1

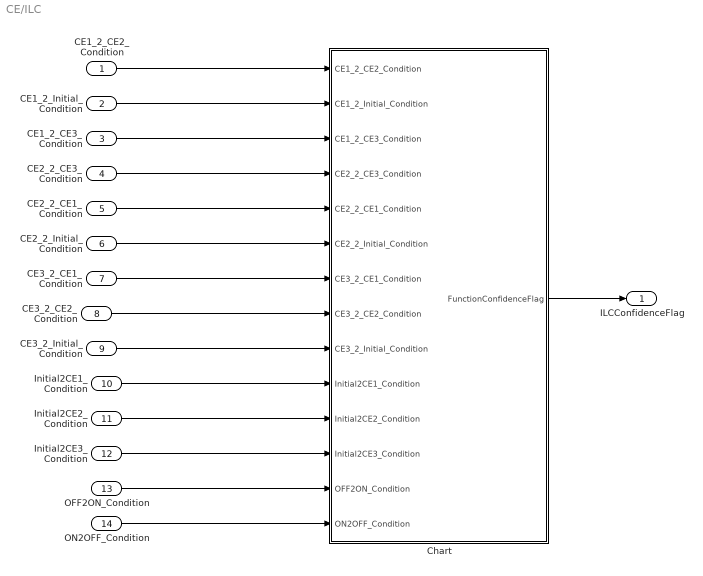
== system CE/ILC ==
  CE1_2_CE2_Condition : Inport
  CE1_2_Initial_Condition : Inport  Port=2
  CE1_2_CE3_Condition : Inport  Port=3
  CE2_2_CE3_Condition : Inport  Port=4
  CE2_2_CE1_Condition : Inport  Port=5
  CE2_2_Initial_Condition : Inport  Port=6
  CE3_2_CE1_Condition : Inport  Port=7
  CE3_2_CE2_Condition : Inport  Port=8
  CE3_2_Initial_Condition : Inport  Port=9
  Initial2CE1_Condition : Inport  Port=10
  Initial2CE2_Condition : Inport  Port=11
  Initial2CE3_Condition : Inport  Port=12
  OFF2ON_Condition : Inport  Port=13
  ON2OFF_Condition : Inport  Port=14
  Chart : Stateflow chart  TreatAsAtomicUnit=on
  ILCConfidenceFlag : Outport
  wires:
  Chart/1(FunctionConfidenceFlag) -> ILCConfidenceFlag/1
  CE1_2_CE2_Condition/1 -> Chart/1(CE1_2_CE2_Condition)
  CE1_2_Initial_Condition/1 -> Chart/2(CE1_2_Initial_Condition)
  CE1_2_CE3_Condition/1 -> Chart/3(CE1_2_CE3_Condition)
  CE2_2_CE3_Condition/1 -> Chart/4(CE2_2_CE3_Condition)
  CE2_2_CE1_Condition/1 -> Chart/5(CE2_2_CE1_Condition)
  CE2_2_Initial_Condition/1 -> Chart/6(CE2_2_Initial_Condition)
  CE3_2_CE1_Condition/1 -> Chart/7(CE3_2_CE1_Condition)
  CE3_2_CE2_Condition/1 -> Chart/8(CE3_2_CE2_Condition)
  CE3_2_Initial_Condition/1 -> Chart/9(CE3_2_Initial_Condition)
  Initial2CE1_Condition/1 -> Chart/10(Initial2CE1_Condition)
  Initial2CE2_Condition/1 -> Chart/11(Initial2CE2_Condition)
  Initial2CE3_Condition/1 -> Chart/12(Initial2CE3_Condition)
  OFF2ON_Condition/1 -> Chart/13(OFF2ON_Condition)
  ON2OFF_Condition/1 -> Chart/14(ON2OFF_Condition)

== system CE/ILCScenarioCodition ==
  In1 : Inport
  ILC_CE1_2_CE2_Condition : Outport
  ILC_CE1_2_Initial_Condition : Outport  Port=2
  ILC_CE1_2_CE3_Condition : Outport  Port=3
  ILC_CE2_2_CE3_Condition : Outport  Port=4
  ILC_CE2_2_CE1_Condition : Outport  Port=5
  ILC_CE2_2_Initial_Condition : Outport  Port=6
  ILC_CE3_2_CE1_Condition : Outport  Port=7
  ILC_CE3_2_CE2_Condition : Outport  Port=8
  ILC_CE3_2_Initial_Condition : Outport  Port=9
  ILC_Initial2CE1_Condition : Outport  Port=10
  ILC_Initial2CE2_Condition : Outport  Port=11
  ILC_Initial2CE3_Condition : Outport  Port=12
  ILC_OFF2ON_Condition : Outport  Port=13
  ILC_ON2OFF_Condition : Outport  Port=14

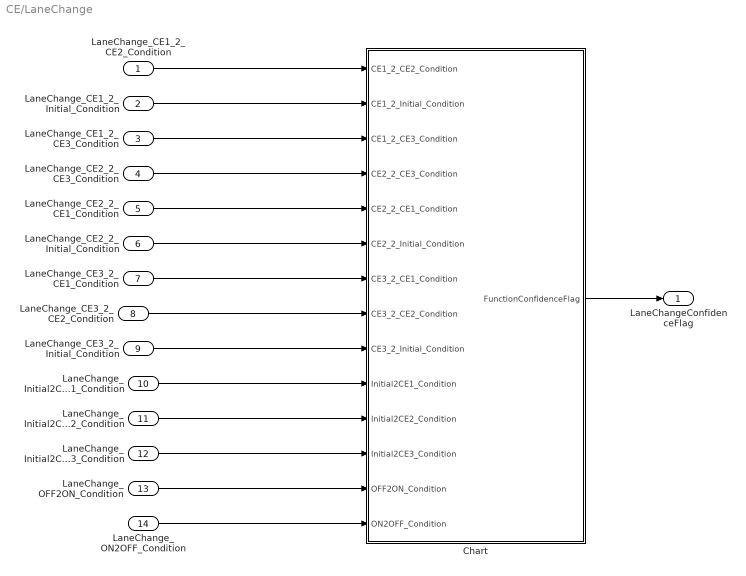
== system CE/LaneChange ==
  LaneChange_CE1_2_CE2_Condition : Inport
  LaneChange_CE1_2_Initial_Condition : Inport  Port=2
  LaneChange_CE1_2_CE3_Condition : Inport  Port=3
  LaneChange_CE2_2_CE3_Condition : Inport  Port=4
  LaneChange_CE2_2_CE1_Condition : Inport  Port=5
  LaneChange_CE2_2_Initial_Condition : Inport  Port=6
  LaneChange_CE3_2_CE1_Condition : Inport  Port=7
  LaneChange_CE3_2_CE2_Condition : Inport  Port=8
  LaneChange_CE3_2_Initial_Condition : Inport  Port=9
  LaneChange_Initial2CE1_Condition : Inport  Port=10
  LaneChange_Initial2CE2_Condition : Inport  Port=11
  LaneChange_Initial2CE3_Condition : Inport  Port=12
  LaneChange_OFF2ON_Condition : Inport  Port=13
  LaneChange_ON2OFF_Condition : Inport  Port=14
  Chart : Stateflow chart  TreatAsAtomicUnit=on
  LaneChangeConfidenceFlag : Outport
  wires:
  LaneChange_ON2OFF_Condition/1 -> Chart/14(ON2OFF_Condition)
  LaneChange_OFF2ON_Condition/1 -> Chart/13(OFF2ON_Condition)
  LaneChange_Initial2CE3_Condition/1 -> Chart/12(Initial2CE3_Condition)
  LaneChange_Initial2CE2_Condition/1 -> Chart/11(Initial2CE2_Condition)
  LaneChange_Initial2CE1_Condition/1 -> Chart/10(Initial2CE1_Condition)
  LaneChange_CE3_2_Initial_Condition/1 -> Chart/9(CE3_2_Initial_Condition)
  LaneChange_CE3_2_CE2_Condition/1 -> Chart/8(CE3_2_CE2_Condition)
  LaneChange_CE3_2_CE1_Condition/1 -> Chart/7(CE3_2_CE1_Condition)
  LaneChange_CE2_2_Initial_Condition/1 -> Chart/6(CE2_2_Initial_Condition)
  LaneChange_CE2_2_CE1_Condition/1 -> Chart/5(CE2_2_CE1_Condition)
  LaneChange_CE2_2_CE3_Condition/1 -> Chart/4(CE2_2_CE3_Condition)
  LaneChange_CE1_2_CE3_Condition/1 -> Chart/3(CE1_2_CE3_Condition)
  LaneChange_CE1_2_Initial_Condition/1 -> Chart/2(CE1_2_Initial_Condition)
  LaneChange_CE1_2_CE2_Condition/1 -> Chart/1(CE1_2_CE2_Condition)
  Chart/1(FunctionConfidenceFlag) -> LaneChangeConfidenceFlag/1

== system CE/LaneChangeScenarioCondition ==
  In1 : Inport
  LaneChange_CE1_2_CE2_Condition : Outport
  LaneChange_CE1_2_Initial_Condition : Outport  Port=2
  LaneChange_CE1_2_CE3_Condition : Outport  Port=3
  LaneChange_CE2_2_CE3_Condition : Outport  Port=4
  LaneChange_CE2_2_CE1_Condition : Outport  Port=5
  LaneChange_CE2_2_Initial_Condition : Outport  Port=6
  LaneChange_CE3_2_CE1_Condition : Outport  Port=7
  LaneChange_CE3_2_CE2_Condition : Outport  Port=8
  LaneChange_CE3_2_Initial_Condition : Outport  Port=9
  LaneChange_Initial2CE1_Condition : Outport  Port=10
  LaneChange_Initial2CE2_Condition : Outport  Port=11
  LaneChange_Initial2CE3_Condition : Outport  Port=12
  LaneChange_OFF2ON_Condition : Outport  Port=13
  LaneChange_ON2OFF_Condition : Outport  Port=14

== system CE/MergeScenarioCodition ==
  In1 : Inport
  Merge_CE1_2_CE2_Condition : Outport
  Merge_CE1_2_Initial_Condition : Outport  Port=2
  Merge_CE1_2_CE3_Condition : Outport  Port=3
  Merge_CE2_2_CE3_Condition : Outport  Port=4
  Merge_CE2_2_CE1_Condition : Outport  Port=5
  Merge_CE2_2_Initial_Condition : Outport  Port=6
  Merge_CE3_2_CE1_Condition : Outport  Port=7
  Merge_CE3_2_CE2_Condition : Outport  Port=8
  Merge_CE3_2_Initial_Condition : Outport  Port=9
  Merge_Initial2CE1_Condition : Outport  Port=10
  Merge_Initial2CE2_Condition : Outport  Port=11
  Merge_Initial2CE3_Condition : Outport  Port=12
  Merge_OFF2ON_Condition : Outport  Port=13
  Merge_ON2OFF_Condition : Outport  Port=14

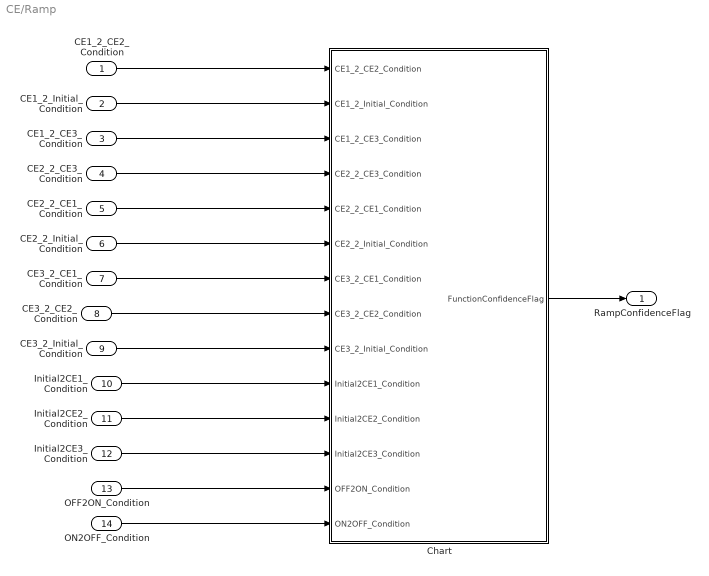
== system CE/Ramp ==
  CE1_2_CE2_Condition : Inport
  CE1_2_Initial_Condition : Inport  Port=2
  CE1_2_CE3_Condition : Inport  Port=3
  CE2_2_CE3_Condition : Inport  Port=4
  CE2_2_CE1_Condition : Inport  Port=5
  CE2_2_Initial_Condition : Inport  Port=6
  CE3_2_CE1_Condition : Inport  Port=7
  CE3_2_CE2_Condition : Inport  Port=8
  CE3_2_Initial_Condition : Inport  Port=9
  Initial2CE1_Condition : Inport  Port=10
  Initial2CE2_Condition : Inport  Port=11
  Initial2CE3_Condition : Inport  Port=12
  OFF2ON_Condition : Inport  Port=13
  ON2OFF_Condition : Inport  Port=14
  Chart : Stateflow chart  TreatAsAtomicUnit=on
  RampConfidenceFlag : Outport
  wires:
  ON2OFF_Condition/1 -> Chart/14(ON2OFF_Condition)
  OFF2ON_Condition/1 -> Chart/13(OFF2ON_Condition)
  Initial2CE3_Condition/1 -> Chart/12(Initial2CE3_Condition)
  Initial2CE2_Condition/1 -> Chart/11(Initial2CE2_Condition)
  Initial2CE1_Condition/1 -> Chart/10(Initial2CE1_Condition)
  CE3_2_Initial_Condition/1 -> Chart/9(CE3_2_Initial_Condition)
  CE3_2_CE2_Condition/1 -> Chart/8(CE3_2_CE2_Condition)
  CE3_2_CE1_Condition/1 -> Chart/7(CE3_2_CE1_Condition)
  CE2_2_Initial_Condition/1 -> Chart/6(CE2_2_Initial_Condition)
  CE2_2_CE1_Condition/1 -> Chart/5(CE2_2_CE1_Condition)
  CE2_2_CE3_Condition/1 -> Chart/4(CE2_2_CE3_Condition)
  CE1_2_CE3_Condition/1 -> Chart/3(CE1_2_CE3_Condition)
  CE1_2_Initial_Condition/1 -> Chart/2(CE1_2_Initial_Condition)
  CE1_2_CE2_Condition/1 -> Chart/1(CE1_2_CE2_Condition)
  Chart/1(FunctionConfidenceFlag) -> RampConfidenceFlag/1

== system CE/RampScenarioCodition ==
  In1 : Inport
  Ramp_CE1_2_CE2_Condition : Outport
  Ramp_CE1_2_Initial_Condition : Outport  Port=2
  Ramp_CE1_2_CE3_Condition : Outport  Port=3
  Ramp_CE2_2_CE3_Condition : Outport  Port=4
  Ramp_CE2_2_CE1_Condition : Outport  Port=5
  Ramp_CE2_2_Initial_Condition : Outport  Port=6
  Ramp_CE3_2_CE1_Condition : Outport  Port=7
  Ramp_CE3_2_CE2_Condition : Outport  Port=8
  Ramp_CE3_2_Initial_Condition : Outport  Port=9
  Ramp_Initial2CE1_Condition : Outport  Port=10
  Ramp_Initial2CE2_Condition : Outport  Port=11
  Ramp_Initial2CE3_Condition : Outport  Port=12
  Ramp_OFF2ON_Condition : Outport  Port=13
  Ramp_ON2OFF_Condition : Outport  Port=14

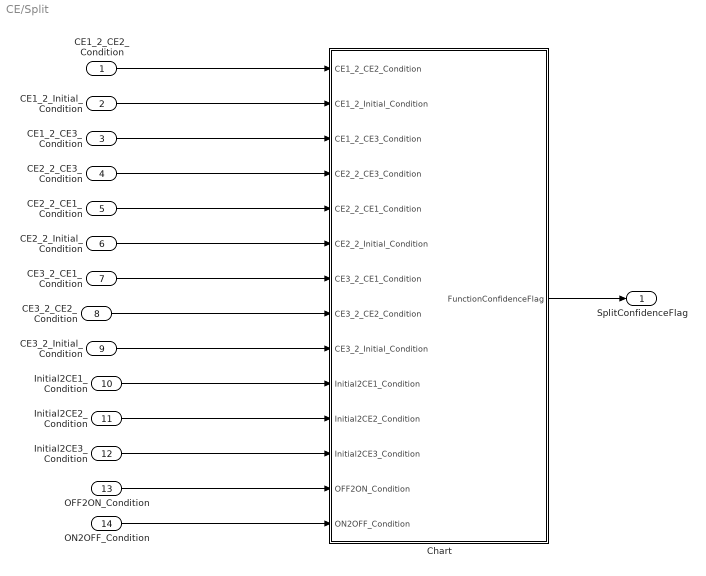
== system CE/Split ==
  CE1_2_CE2_Condition : Inport
  CE1_2_Initial_Condition : Inport  Port=2
  CE1_2_CE3_Condition : Inport  Port=3
  CE2_2_CE3_Condition : Inport  Port=4
  CE2_2_CE1_Condition : Inport  Port=5
  CE2_2_Initial_Condition : Inport  Port=6
  CE3_2_CE1_Condition : Inport  Port=7
  CE3_2_CE2_Condition : Inport  Port=8
  CE3_2_Initial_Condition : Inport  Port=9
  Initial2CE1_Condition : Inport  Port=10
  Initial2CE2_Condition : Inport  Port=11
  Initial2CE3_Condition : Inport  Port=12
  OFF2ON_Condition : Inport  Port=13
  ON2OFF_Condition : Inport  Port=14
  Chart : Stateflow chart  TreatAsAtomicUnit=on
  SplitConfidenceFlag : Outport
  wires:
  Chart/1(FunctionConfidenceFlag) -> SplitConfidenceFlag/1
  CE1_2_CE2_Condition/1 -> Chart/1(CE1_2_CE2_Condition)
  CE1_2_Initial_Condition/1 -> Chart/2(CE1_2_Initial_Condition)
  CE1_2_CE3_Condition/1 -> Chart/3(CE1_2_CE3_Condition)
  CE2_2_CE3_Condition/1 -> Chart/4(CE2_2_CE3_Condition)
  CE2_2_CE1_Condition/1 -> Chart/5(CE2_2_CE1_Condition)
  CE2_2_Initial_Condition/1 -> Chart/6(CE2_2_Initial_Condition)
  CE3_2_CE1_Condition/1 -> Chart/7(CE3_2_CE1_Condition)
  CE3_2_CE2_Condition/1 -> Chart/8(CE3_2_CE2_Condition)
  CE3_2_Initial_Condition/1 -> Chart/9(CE3_2_Initial_Condition)
  Initial2CE1_Condition/1 -> Chart/10(Initial2CE1_Condition)
  Initial2CE2_Condition/1 -> Chart/11(Initial2CE2_Condition)
  Initial2CE3_Condition/1 -> Chart/12(Initial2CE3_Condition)
  OFF2ON_Condition/1 -> Chart/13(OFF2ON_Condition)
  ON2OFF_Condition/1 -> Chart/14(ON2OFF_Condition)

== system CE/SplitScenarioCodition ==
  In1 : Inport
  Split_CE1_2_CE2_Condition : Outport
  Split_CE1_2_Initial_Condition : Outport  Port=2
  Split_CE1_2_CE3_Condition : Outport  Port=3
  Split_CE2_2_CE3_Condition : Outport  Port=4
  Split_CE2_2_CE1_Condition : Outport  Port=5
  Split_CE2_2_Initial_Condition : Outport  Port=6
  Split_CE3_2_CE1_Condition : Outport  Port=7
  Split_CE3_2_CE2_Condition : Outport  Port=8
  Split_CE3_2_Initial_Condition : Outport  Port=9
  Split_Initial2CE1_Condition : Outport  Port=10
  Split_Initial2CE2_Condition : Outport  Port=11
  Split_Initial2CE3_Condition : Outport  Port=12
  Split_OFF2ON_Condition : Outport  Port=13
  Split_ON2OFF_Condition : Outport  Port=14

== system CE/TrafficDencity ==
  SDF_Object : Inport
  Chart : Stateflow chart  TreatAsAtomicUnit=on
  TrafficDencity : Outport
  wires:
  SDF_Object/1 -> Chart/1(SDF_Object)
  Chart/1(TrafficDencity) -> TrafficDencity/1

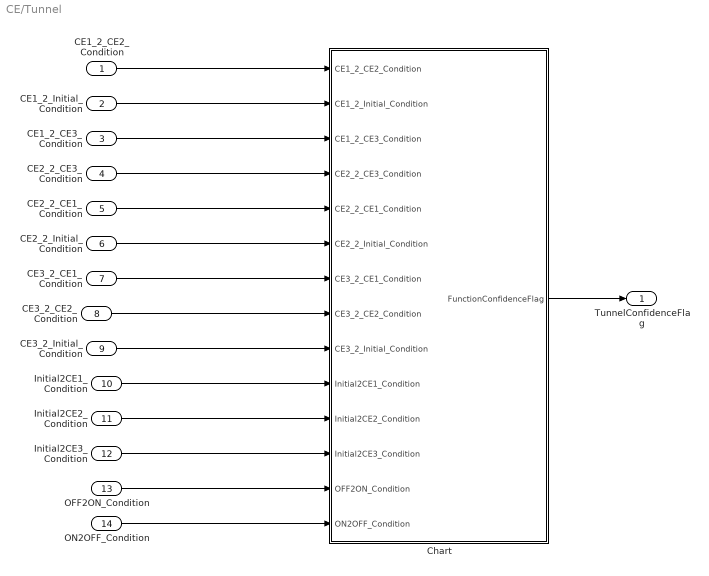
== system CE/Tunnel ==
  CE1_2_CE2_Condition : Inport
  CE1_2_Initial_Condition : Inport  Port=2
  CE1_2_CE3_Condition : Inport  Port=3
  CE2_2_CE3_Condition : Inport  Port=4
  CE2_2_CE1_Condition : Inport  Port=5
  CE2_2_Initial_Condition : Inport  Port=6
  CE3_2_CE1_Condition : Inport  Port=7
  CE3_2_CE2_Condition : Inport  Port=8
  CE3_2_Initial_Condition : Inport  Port=9
  Initial2CE1_Condition : Inport  Port=10
  Initial2CE2_Condition : Inport  Port=11
  Initial2CE3_Condition : Inport  Port=12
  OFF2ON_Condition : Inport  Port=13
  ON2OFF_Condition : Inport  Port=14
  Chart : Stateflow chart  TreatAsAtomicUnit=on
  TunnelConfidenceFlag : Outport
  wires:
  ON2OFF_Condition/1 -> Chart/14(ON2OFF_Condition)
  OFF2ON_Condition/1 -> Chart/13(OFF2ON_Condition)
  Initial2CE3_Condition/1 -> Chart/12(Initial2CE3_Condition)
  Initial2CE2_Condition/1 -> Chart/11(Initial2CE2_Condition)
  Initial2CE1_Condition/1 -> Chart/10(Initial2CE1_Condition)
  CE3_2_Initial_Condition/1 -> Chart/9(CE3_2_Initial_Condition)
  CE3_2_CE2_Condition/1 -> Chart/8(CE3_2_CE2_Condition)
  CE3_2_CE1_Condition/1 -> Chart/7(CE3_2_CE1_Condition)
  CE2_2_Initial_Condition/1 -> Chart/6(CE2_2_Initial_Condition)
  CE2_2_CE1_Condition/1 -> Chart/5(CE2_2_CE1_Condition)
  CE2_2_CE3_Condition/1 -> Chart/4(CE2_2_CE3_Condition)
  CE1_2_CE3_Condition/1 -> Chart/3(CE1_2_CE3_Condition)
  CE1_2_Initial_Condition/1 -> Chart/2(CE1_2_Initial_Condition)
  CE1_2_CE2_Condition/1 -> Chart/1(CE1_2_CE2_Condition)
  Chart/1(FunctionConfidenceFlag) -> TunnelConfidenceFlag/1

== system CE/TunnelScenarioCodition ==
  In1 : Inport
  Tunnel_CE1_2_CE2_Condition : Outport
  Tunnel_CE1_2_Initial_Condition : Outport  Port=2
  Tunnel_CE1_2_CE3_Condition : Outport  Port=3
  Tunnel_CE2_2_CE3_Condition : Outport  Port=4
  Tunnel_CE2_2_CE1_Condition : Outport  Port=5
  Tunnel_CE2_2_Initial_Condition : Outport  Port=6
  Tunnel_CE3_2_CE1_Condition : Outport  Port=7
  Tunnel_CE3_2_CE2_Condition : Outport  Port=8
  Tunnel_CE3_2_Initial_Condition : Outport  Port=9
  Tunnel_Initial2CE1_Condition : Outport  Port=10
  Tunnel_Initial2CE2_Condition : Outport  Port=11
  Tunnel_Initial2CE3_Condition : Outport  Port=12
  Tunnel_OFF2ON_Condition : Outport  Port=13
  LaneChange_ON2OFF_Condition : Outport  Port=14

== system CE/WrapperCE ==
  In1 : Inport
  Out1 : Outport
  Out2 : Outport  Port=2
  Out3 : Outport  Port=3
  Out4 : Outport  Port=4
